simulink model "LQ_control"  (R2022a)
settings: Solver=VariableStepAuto  StartTime=0.0  StopTime=5  RelTol=1e-3
values from neighbouring files (symbols this model uses):
  Ad = ss_d.A    [ControllerwithDelay.m]    (also in ControllerwithDelay_LQR.m; ControllerwithDelay_PID.m; ControllerwithDelay_SS.m; DiscreteLQControl.m)
  Bd = ss_d.B    [ControllerwithDelay.m]    (also in ControllerwithDelay_LQR.m; ControllerwithDelay_PID.m; ControllerwithDelay_SS.m; DiscreteLQControl.m)
  Cd = ss_d.C    [ControllerwithDelay.m]    (also in ControllerwithDelay_LQR.m; ControllerwithDelay_PID.m; ControllerwithDelay_SS.m; DiscreteLQControl.m)
  K2 = [10.6418, 0.6377,0.0143,1]    [steadyStateError.m]
undefined symbols (not defined in the file or in its folder): K1, K3, K4, K5, K6
settings Model: Creator=1  LastModifiedBy=1

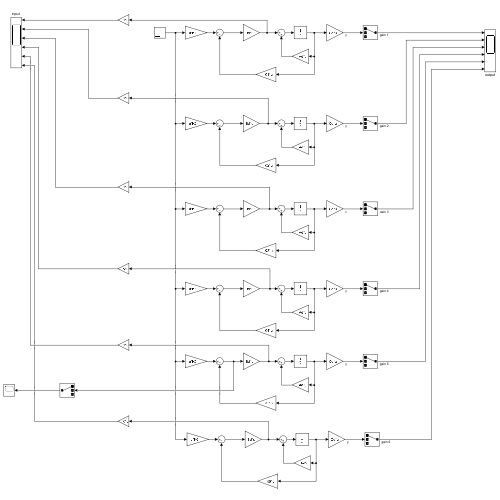
[thumbnail: Simulink's stored preview of the top-level diagram]
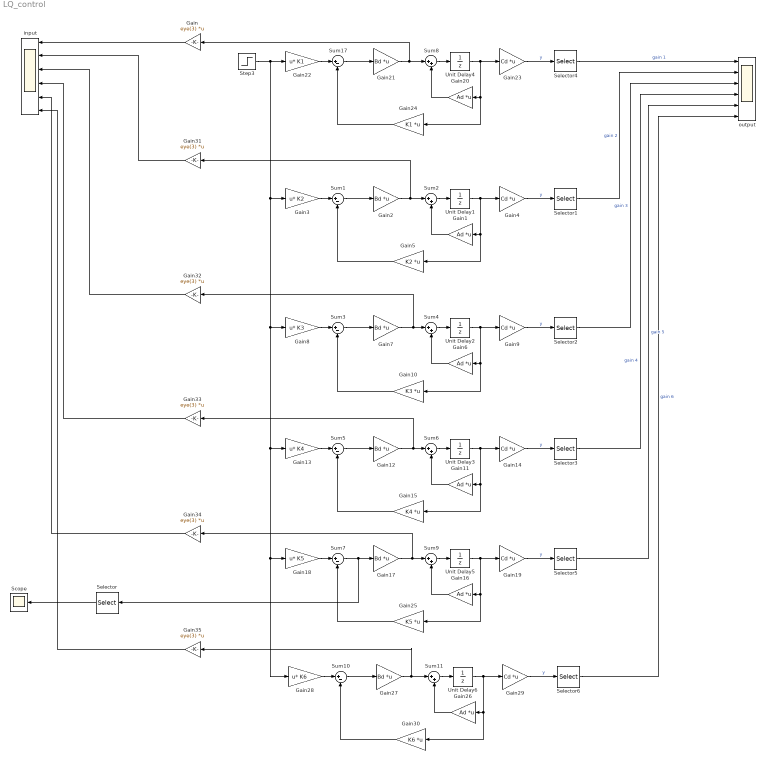
== system LQ_control ==
  Gain{,31..35} (6 alike) : Gain  Gain=eye(3)  Multiplication=Matrix(K*u)
  Gain{1,6,11,16,20,26} (6 alike) : Gain  Gain=Ad  Multiplication=Matrix(K*u)
  Gain10 : Gain  Gain=K3  Multiplication=Matrix(K*u)
  Gain{2,7,12,17,21,27} (6 alike) : Gain  Gain=Bd  Multiplication=Matrix(K*u)
  Gain13 : Gain  Gain=K4  Multiplication=Matrix(u*K)
  Gain{4,9,14,19,23,29} (6 alike) : Gain  Gain=Cd  Multiplication=Matrix(K*u)
  Gain15 : Gain  Gain=K4  Multiplication=Matrix(K*u)
  Gain18 : Gain  Gain=K5  Multiplication=Matrix(u*K)
  Gain22 : Gain  Gain=K1  Multiplication=Matrix(u*K)
  Gain24 : Gain  Gain=K1  Multiplication=Matrix(K*u)
  Gain25 : Gain  Gain=K5  Multiplication=Matrix(K*u)
  Gain28 : Gain  Gain=K6  Multiplication=Matrix(u*K)
  Gain3 : Gain  Gain=K2  Multiplication=Matrix(u*K)
  Gain30 : Gain  Gain=K6  Multiplication=Matrix(K*u)
  Gain5 : Gain  Gain=K2  Multiplication=Matrix(K*u)
  Gain8 : Gain  Gain=K3  Multiplication=Matrix(u*K)
  Scope : Scope
  Selector{,1..6} (7 alike) : Selector  InputPortWidth=3  IndexOptions=Index vector (dialog)  Indices=[1]  OutputSizes=1
  Step3 : Step  Time=0.1  SampleTime=0
  Sum{1,3,5,7,10,17} (6 alike) : Sum  Inputs=|+-
  Sum{2,4,6,8..9,11} (6 alike) : Sum  Inputs=|++
  Unit Delay{1..6} (6 alike) : UnitDelay  SampleTime=-1  HasFrameUpgradeWarning=on
  "input " : Scope  NumInputPorts=6
  output : Scope  NumInputPorts=6
  wires:
  Gain20/1 -> Sum8/2
  Gain24/1 -> Sum17/2
  Sum17/1 -> Gain21/1
  Gain22/1 -> Sum17/1
  Gain23/1 -> Selector4/1  "y"
  Step3/1 -> Gain8/1, Gain28/1, Gain18/1, Gain13/1, Gain3/1, Gain22/1
  Unit Delay4/1 -> Gain20/1, Gain24/1, Gain23/1
  Sum8/1 -> Unit Delay4/1
  Gain21/1 -> Gain/1, Sum8/1
  Selector4/1 -> output/1  "gain 1"
  Gain1/1 -> Sum2/2
  Gain2/1 -> Gain31/1, Sum2/1
  Unit Delay1/1 -> Gain1/1, Gain5/1, Gain4/1
  Sum1/1 -> Gain2/1
  Gain4/1 -> Selector1/1  "y"
  Gain3/1 -> Sum1/1
  Gain5/1 -> Sum1/2
  Sum2/1 -> Unit Delay1/1
  Sum4/1 -> Unit Delay2/1
  Gain10/1 -> Sum3/2
  Sum3/1 -> Gain7/1
  Gain9/1 -> Selector2/1  "y"
  Gain7/1 -> Gain32/1, Sum4/1
  Gain8/1 -> Sum3/1
  Unit Delay2/1 -> Gain6/1, Gain10/1, Gain9/1
  Gain6/1 -> Sum4/2
  Sum6/1 -> Unit Delay3/1
  Gain15/1 -> Sum5/2
  Sum5/1 -> Gain12/1
  Gain14/1 -> Selector3/1  "y"
  Gain12/1 -> Gain33/1, Sum6/1
  Gain13/1 -> Sum5/1
  Unit Delay3/1 -> Gain11/1, Gain15/1, Gain14/1
  Gain11/1 -> Sum6/2
  Sum9/1 -> Unit Delay5/1
  Gain25/1 -> Sum7/2
  Sum7/1 -> Selector/1, Gain17/1
  Gain19/1 -> Selector5/1  "y"
  Gain18/1 -> Sum7/1
  Unit Delay5/1 -> Gain16/1, Gain25/1, Gain19/1
  Gain16/1 -> Sum9/2
  Sum11/1 -> Unit Delay6/1
  Gain30/1 -> Sum10/2
  Sum10/1 -> Gain27/1
  Gain29/1 -> Selector6/1  "y"
  Gain27/1 -> Gain35/1, Sum11/1
  Gain28/1 -> Sum10/1
  Unit Delay6/1 -> Gain26/1, Gain30/1, Gain29/1
  Gain26/1 -> Sum11/2
  Selector1/1 -> output/2  "gain 2"
  Selector2/1 -> output/3  "gain 3"
  Selector3/1 -> output/4  "gain 4"
  Selector5/1 -> output/5  "gain 5"
  Selector6/1 -> output/6  "gain 6"
  Gain17/1 -> Sum9/1, Gain34/1
  Gain/1 -> "input "/1
  Gain31/1 -> "input "/2
  Gain32/1 -> "input "/3
  Gain33/1 -> "input "/4
  Gain35/1 -> "input "/6
  Gain34/1 -> "input "/5
  Selector/1 -> Scope/1
